simulink model "ReflexiveInhibition"  (Simulink 7.1)
settings: Solver=ode45  StartTime=0.0  StopTime=1  RelTol=1e-3
libraries: NeuroModelerLibrary x17
settings Model: Creator=Bakhshiev  LastModifiedBy=Bakhshiev

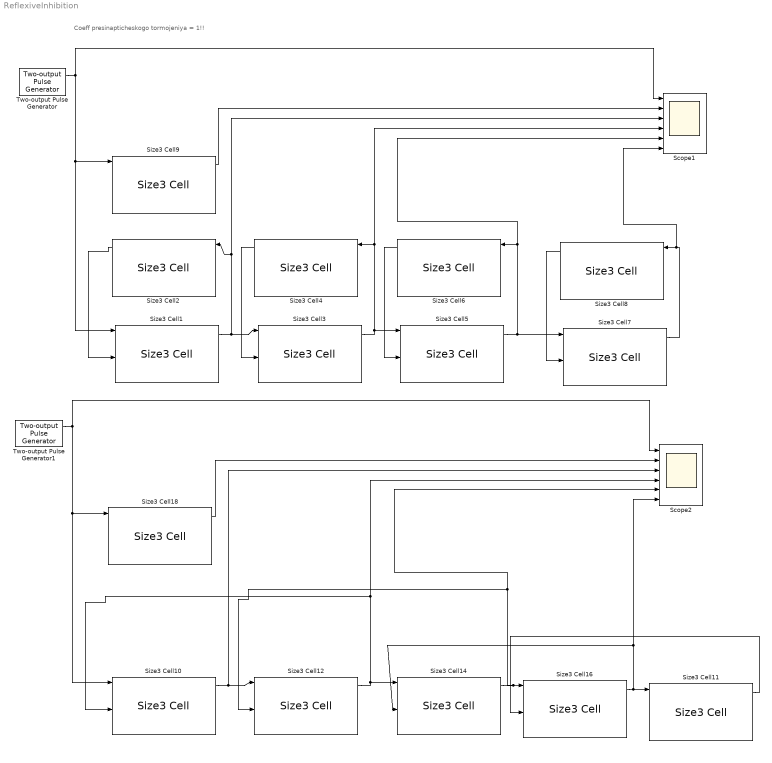
== system ReflexiveInhibition ==
  note: Coeff presinapticheskogo tormojeniya = 1!!
  Scope1 : Scope  NumInputPorts=6
      settings: TimeRange=1  YMin=0~0~0~0~0~0  YMax=1~1~1~1~1~1  MaxDataPoints=5000000
  Scope2 : Scope  NumInputPorts=6
      settings: TimeRange=1  YMin=0~0~0~0~0~0  YMax=1~1~1~1~1~1  MaxDataPoints=5000000
  Size3 Cell1 : NeuroModelerLibrary/Sized Cells/Size3 Cell  SystemSampleTime=-1
      link override Synapse2: ksi=1
      link override Synapse3: ksi=1
  Size3 Cell10 : NeuroModelerLibrary/Sized Cells/Size3 Cell  SystemSampleTime=-1
      link override Synapse2: ksi=1
      link override Synapse3: ksi=1
  Size3 Cell11 : NeuroModelerLibrary/Sized Cells/Size3 Cell  SystemSampleTime=-1
      link override Synapse2: ksi=1
      link override Synapse3: ksi=1
  Size3 Cell12 : NeuroModelerLibrary/Sized Cells/Size3 Cell  SystemSampleTime=-1
      link override Synapse2: ksi=1
      link override Synapse3: ksi=1
  Size3 Cell14 : NeuroModelerLibrary/Sized Cells/Size3 Cell  SystemSampleTime=-1
      link override Synapse2: ksi=1
      link override Synapse3: ksi=1
  Size3 Cell16 : NeuroModelerLibrary/Sized Cells/Size3 Cell  SystemSampleTime=-1
      link override Synapse2: ksi=1
      link override Synapse3: ksi=1
  Size3 Cell18 : NeuroModelerLibrary/Sized Cells/Size3 Cell  SystemSampleTime=-1
      link override Synapse2: ksi=1
      link override Synapse3: ksi=1
  Size3 Cell2 : NeuroModelerLibrary/Sized Cells/Size3 Cell  Orientation=left  SystemSampleTime=-1
      link override Synapse2: ksi=1
      link override Synapse3: ksi=1
  Size3 Cell3 : NeuroModelerLibrary/Sized Cells/Size3 Cell  SystemSampleTime=-1
      link override Synapse2: ksi=1
      link override Synapse3: ksi=1
  Size3 Cell4 : NeuroModelerLibrary/Sized Cells/Size3 Cell  Orientation=left  SystemSampleTime=-1
      link override Synapse2: ksi=1
      link override Synapse3: ksi=1
  Size3 Cell5 : NeuroModelerLibrary/Sized Cells/Size3 Cell  SystemSampleTime=-1
      link override Synapse2: ksi=1
      link override Synapse3: ksi=1
  Size3 Cell6 : NeuroModelerLibrary/Sized Cells/Size3 Cell  Orientation=left  SystemSampleTime=-1
      link override Synapse2: ksi=1
      link override Synapse3: ksi=1
  Size3 Cell7 : NeuroModelerLibrary/Sized Cells/Size3 Cell  SystemSampleTime=-1
      link override Synapse2: ksi=1
      link override Synapse3: ksi=1
  Size3 Cell8 : NeuroModelerLibrary/Sized Cells/Size3 Cell  Orientation=left  SystemSampleTime=-1
      link override Synapse2: ksi=1
      link override Synapse3: ksi=1
  Size3 Cell9 : NeuroModelerLibrary/Sized Cells/Size3 Cell  SystemSampleTime=-1
      link override Synapse2: ksi=1
      link override Synapse3: ksi=1
  Two-output Pulse Generator : NeuroModelerLibrary/Support/Two-output Pulse Generator  SystemSampleTime=-1  A=1  P1=40  P2=200  PW=1  ST=0.001  OOn1=0.15  OOff1=1  OOn2=0.25  OOff2=0.3
  Two-output Pulse Generator1 : NeuroModelerLibrary/Support/Two-output Pulse Generator  SystemSampleTime=-1  A=1  P1=40  P2=200  PW=1  ST=0.001  OOn1=0.15  OOff1=1  OOn2=0.25  OOff2=0.3
  wires:
  Two-output Pulse Generator/1 -> Size3 Cell1/1, Size3 Cell9/1, Scope1/1
  Size3 Cell1/1 -> Size3 Cell3/1, Size3 Cell2/1, Scope1/3
  Size3 Cell2/1 -> Size3 Cell1/5
  Size3 Cell4/1 -> Size3 Cell3/5
  Size3 Cell3/1 -> Size3 Cell4/1, Scope1/4, Size3 Cell5/1
  Size3 Cell6/1 -> Size3 Cell5/5
  Size3 Cell5/1 -> Size3 Cell6/1, Scope1/5, Size3 Cell7/1
  Size3 Cell8/1 -> Size3 Cell7/5
  Size3 Cell7/1 -> Size3 Cell8/1, Scope1/6
  Size3 Cell9/1 -> Scope1/2
  Two-output Pulse Generator1/1 -> Size3 Cell10/1, Size3 Cell18/1, Scope2/1
  Size3 Cell10/1 -> Size3 Cell12/1, Scope2/3
  Size3 Cell12/1 -> Scope2/4, Size3 Cell10/5, Size3 Cell14/1
  Size3 Cell14/1 -> Scope2/5, Size3 Cell12/5, Size3 Cell16/1
  Size3 Cell18/1 -> Scope2/2
  Size3 Cell16/1 -> Size3 Cell11/1, Size3 Cell14/5, Scope2/6
  Size3 Cell11/1 -> Size3 Cell16/5
